simulink model "series_rlc_model"  (R2024a)
settings: Solver=VariableStepAuto  StartTime=0.0  StopTime=0.5  RelTol=1e-3
undefined symbols (not defined in the file): C_val, L_val, R_val, w_0
settings Model: Creator=asafi  LastModifiedBy=asafhayon
settings ConfigComp: CovBoundaryAbsTol=1.0e-5

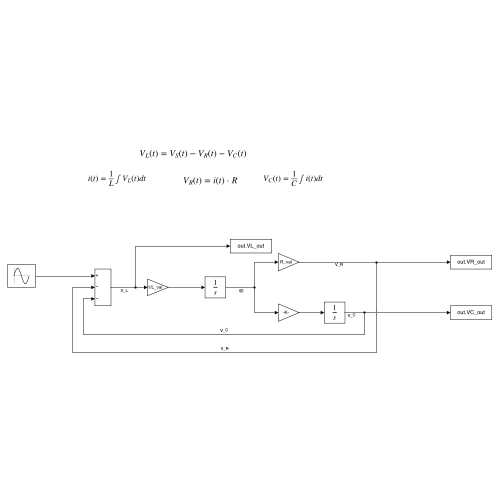
[thumbnail: Simulink's stored preview of the top-level diagram]
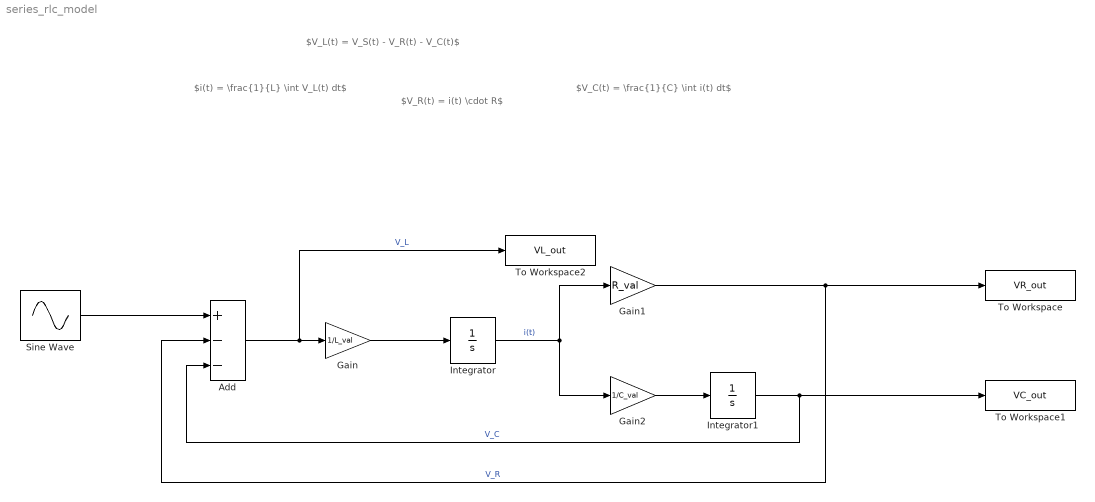
== system series_rlc_model ==
  note: $V_C(t) = \frac{1}{C} \int i(t) dt$
  note: $V_R(t) = i(t) \cdot R$
  note: $i(t) = \frac{1}{L} \int V_L(t) dt$
  note: $V_L(t) = V_S(t) - V_R(t) - V_C(t)$
  Add : Sum  Inputs=+--
  Gain : Gain  Gain=1/L_val
  Gain1 : Gain  Gain=R_val
  Gain2 : Gain  Gain=1/C_val
  Integrator : Integrator
  Integrator1 : Integrator
  Sine Wave : Sin  Frequency=w_0  Phase=pi/2  SampleTime=0
  To Workspace : ToWorkspace  VariableName=VR_out  SampleTime=-1
  To Workspace1 : ToWorkspace  VariableName=VC_out  SampleTime=-1
  To Workspace2 : ToWorkspace  VariableName=VL_out  SampleTime=-1
  wires:
  Sine Wave/1 -> Add/1
  Add/1 -> To Workspace2/1, Gain/1  "V_L"
  Gain/1 -> Integrator/1
  Integrator/1 -> Gain2/1, Gain1/1  "i(t)"
  Gain2/1 -> Integrator1/1
  Integrator1/1 -> To Workspace1/1, Add/3  "V_C"
  Gain1/1 -> To Workspace/1, Add/2  "V_R"
